simulink model "NonLiniarModel"  (R2023a)
settings: Solver=ode4  StartTime=0.0  StopTime=run_time  FixedStep=0.01  RelTol=1e-3
values from neighbouring files (symbols this model uses):
  g = 9.81    [PreLab.m]    (also in PreLab_for_lab.m)
  l = 0.35    [PreLab.m]    (also in PreLab_for_lab.m)
  m = 0.04    [PreLab.m]    (also in PreLab_for_lab.m)
  Myu_d = 1.3*10^(-4)    (= 0.00013)    [PreLab.m]    (also in PreLab_for_lab.m)
  Myu_v = 6.7*10^(-5)    (= 6.7e-05)    [PreLab.m]    (also in PreLab_for_lab.m)
  theta_0 = initial_theta_rad(i)    [PreLab.m]    (also in PreLab_for_lab.m)
  theta_dot_0 = 0    [PreLab.m]    (also in PreLab_for_lab.m)
settings Model: Creator=אלמוג  LastModifiedBy=אלמוג

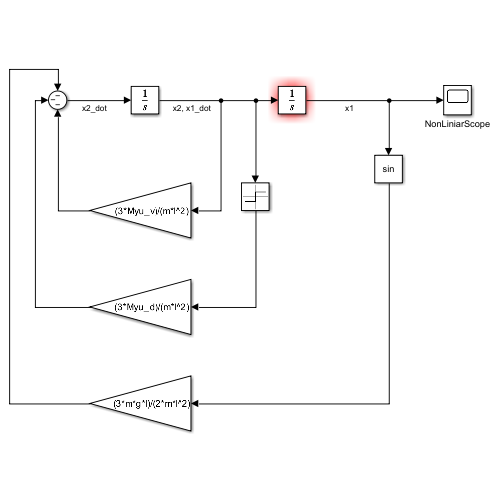
[thumbnail: Simulink's stored preview of the top-level diagram]
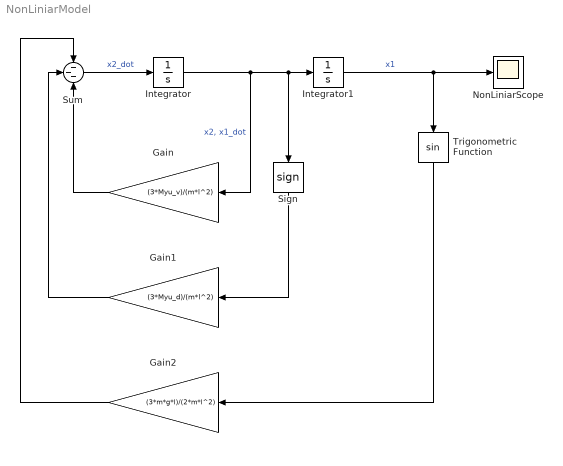
== system NonLiniarModel ==
  Gain : Gain  Gain=(3*Myu_v)/(m*l^2)
  Gain1 : Gain  Gain=(3*Myu_d)/(m*l^2)
  Gain2 : Gain  Gain=(3*m*g*l)/(2*m*l^2)
  Integrator : Integrator  InitialCondition=theta_dot_0
  Integrator1 : Integrator  InitialCondition=theta_0
  NonLiniarScope : Scope
  Sign : Signum
  Sum : Sum  Inputs=---
  Trigonometric Function : Trigonometry
  wires:
  Integrator/1 -> Gain/1, Sign/1, Integrator1/1  "x2, x1_dot"
  Sum/1 -> Integrator/1  "x2_dot"
  Integrator1/1 -> NonLiniarScope/1, Trigonometric Function/1  "x1"
  Sign/1 -> Gain1/1
  Trigonometric Function/1 -> Gain2/1
  Gain/1 -> Sum/3
  Gain1/1 -> Sum/2
  Gain2/1 -> Sum/1
